simulink model "MCCULLOUGH_Andrew_Proj4_simulink"  (R2018b)
settings: Solver=FixedStepDiscrete  StartTime=0.0  StopTime=0.1  FixedStep=1e-7  RelTol=1e-3
libraries: powerlib x20, simulink x1
settings Model: Creator=Andrew McCullough  LastModifiedBy=Andrew McCullough

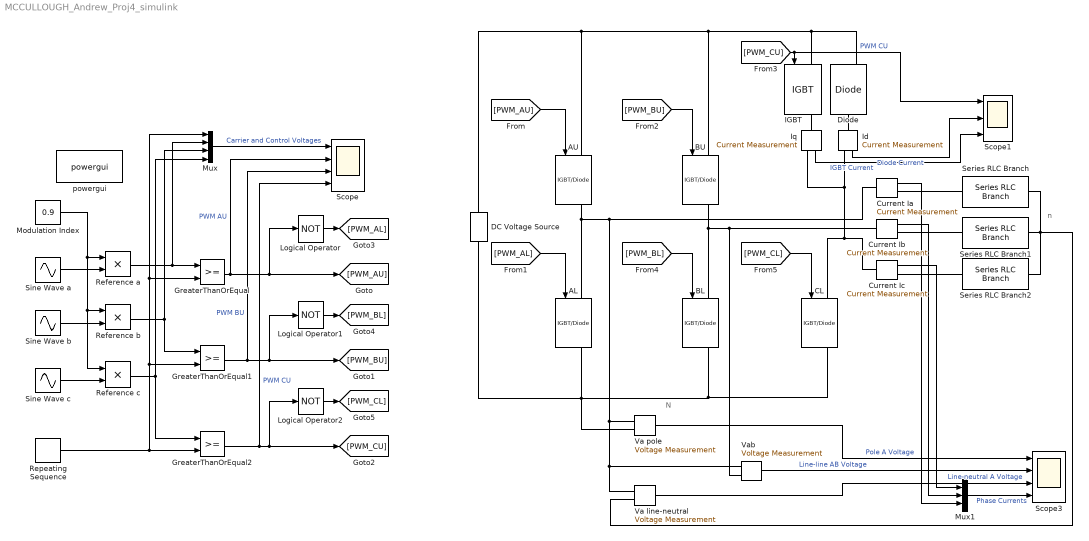
== system MCCULLOUGH_Andrew_Proj4_simulink ==
  note: n
  note: N
  AL : powerlib/Power Electronics/IGBT//Diode  Ron=1e-3  Rs=1e5  Cs=inf  Measurements=on
  AU : powerlib/Power Electronics/IGBT//Diode  Ron=1e-3  Rs=1e5  Cs=inf  Measurements=on
  BL : powerlib/Power Electronics/IGBT//Diode  Ron=1e-3  Rs=1e5  Cs=inf  Measurements=on
  BU : powerlib/Power Electronics/IGBT//Diode  Ron=1e-3  Rs=1e5  Cs=inf  Measurements=on
  CL : powerlib/Power Electronics/IGBT//Diode  Ron=1e-3  Rs=1e5  Cs=inf  Measurements=on
  Current Ia : powerlib/Measurements/Current Measurement  PhasorSimulation=off  OutputType=Complex  PSBequivalent=0
  Current Ib : powerlib/Measurements/Current Measurement  PhasorSimulation=off  OutputType=Complex  PSBequivalent=0
  Current Ic : powerlib/Measurements/Current Measurement  PhasorSimulation=off  OutputType=Complex  PSBequivalent=0
  DC Voltage Source : powerlib/Electrical Sources/DC Voltage Source  Amplitude=400  Measurements=None
  Diode : powerlib/Power Electronics/Diode  Ron=0.001  Lon=0  Vf=0.8  IC=0  UseSnubber=0  Rs=500  Cs=250e-9  Measurements=on
  GreaterThanOrEqual : RelationalOperator  OutDataTypeStr=boolean  RndMeth=Simplest
  GreaterThanOrEqual1 : RelationalOperator  OutDataTypeStr=boolean  RndMeth=Simplest
  GreaterThanOrEqual2 : RelationalOperator  OutDataTypeStr=boolean  RndMeth=Simplest
  IGBT : powerlib/Power Electronics/IGBT  Ron=0.001  Lon=0  Vf=1  Tf=1e-6  Tt=2e-6  IC=0  Rs=1e5  Cs=inf  Measurements=on
  Id : powerlib/Measurements/Current Measurement  PhasorSimulation=off  OutputType=Complex  PSBequivalent=0
  Iq : powerlib/Measurements/Current Measurement  PhasorSimulation=off  OutputType=Complex  PSBequivalent=0
  Logical Operator : Logic  Operator=NOT  AllPortsSameDT=off  OutDataTypeStr=boolean
  Logical Operator1 : Logic  Operator=NOT  AllPortsSameDT=off  OutDataTypeStr=boolean
  Logical Operator2 : Logic  Operator=NOT  AllPortsSameDT=off  OutDataTypeStr=boolean
  Modulation Index : Constant  Value=0.9
  Mux : Mux
  Mux1 : Mux  Inputs=3
  Reference a : Product
  Reference b : Product
  Reference c : Product
  Repeating Sequence : simulink/Sources/Repeating Sequence  rep_seq_t=[0 ((1/2)*(1/15000)) (1/15000)]  rep_seq_y=[-1 1 -1]
  Scope : Scope  NumInputPorts=4
  Scope1 : Scope  NumInputPorts=3
  Scope3 : Scope  NumInputPorts=4
  Series RLC Branch : powerlib/Elements/Series RLC Branch  LConnTagsString=__new0  RConnTagsString=__new0  BranchType=RL  Resistance=.3  Inductance=0.2e-3  SetiL0=off  InitialCurrent=0  Capacitance=0  Setx0=off  InitialVoltage=0  Measurements=None
  Series RLC Branch1 : powerlib/Elements/Series RLC Branch  LConnTagsString=__new0  RConnTagsString=__new0  BranchType=RL  Resistance=.3  Inductance=0.2e-3  SetiL0=off  InitialCurrent=0  Capacitance=0  Setx0=off  InitialVoltage=0  Measurements=None
  Series RLC Branch2 : powerlib/Elements/Series RLC Branch  LConnTagsString=__new0  RConnTagsString=__new0  BranchType=RL  Resistance=.3  Inductance=0.2e-3  SetiL0=off  InitialCurrent=0  Capacitance=0  Setx0=off  InitialVoltage=0  Measurements=None
  Sine Wave a : Sin  Frequency=2*100*pi  SampleTime=0
  Sine Wave b : Sin  Frequency=2*100*pi  Phase=120*(pi/180)  SampleTime=0
  Sine Wave c : Sin  Frequency=2*100*pi  Phase=-120*(pi/180)  SampleTime=0
  Va line-neutral : powerlib/Measurements/Voltage Measurement  PhasorSimulation=off  OutputType=Complex  PSBequivalent=0
  Va pole : powerlib/Measurements/Voltage Measurement  PhasorSimulation=off  OutputType=Complex  PSBequivalent=0
  Vab : powerlib/Measurements/Voltage Measurement  PhasorSimulation=off  OutputType=Complex  PSBequivalent=0
  powergui : powerlib/powergui  Priority=1  SimulationMode=Discrete  SampleTime=1e-7  frequency=60  Iterations=50  frequencyindice=0  Pbase=100e6  ErrMax=1e-4  UnitsV=kV  UnitsW=MW  buscounter=0  FunctionMessages=off  echomessages=off  EnableUseOfTLC=off  CurrentSourceSwitches=off  DisableSnubberDevices=off  DisableRonSwitches=off  DisableVfSwitches=off  DisplayEquations=off  SolverType=Tustin/Backward Euler (TBE)  Interpol=off  ExternalGateDelay=off  methode=off  Ts=100  x0status=blocks  SPID=off  SwTol=0  HookPort=off  RestoreLinks=warning  ResistiveCurrentMeasurement=off  Frange=[0:2:500]  Ylog=off  Xlog=on  ShowGrid=off  save=off  variable=ZData  structure=0  ZoomFFT=off  StartTime=0.0  cycles=1  DisplayStyle=1  fundamental=60  FreqAxis=off  MaxFrequency=1000  frequencyindicesteady=1  RmsSteady=1  display=off
  wires:
  Sine Wave a/1 -> Reference a/2
  Sine Wave b/1 -> Reference b/2
  Sine Wave c/1 -> Reference c/2
  Modulation Index/1 -> Reference a/1, Reference b/1, Reference c/1
  Reference a/1 -> GreaterThanOrEqual/1, Mux/2
  Reference b/1 -> GreaterThanOrEqual1/1, Mux/3
  Reference c/1 -> GreaterThanOrEqual2/1, Mux/4
  Repeating Sequence/1 -> Mux/1, GreaterThanOrEqual/2, GreaterThanOrEqual1/2, GreaterThanOrEqual2/2
  GreaterThanOrEqual2/1 -> Logical Operator2/1, [PWM_CU], Scope/4  "PWM CU"
  GreaterThanOrEqual1/1 -> Logical Operator1/1, [PWM_BU], Scope/3  "PWM BU"
  GreaterThanOrEqual/1 -> [PWM_AU], Logical Operator/1, Scope/2  "PWM AU"
  Logical Operator/1 -> [PWM_AL]
  Logical Operator1/1 -> [PWM_BL]
  Logical Operator2/1 -> [PWM_CL]
  Mux/1 -> Scope/1  "Carrier and Control Voltages"
  [PWM_AU] -> AU/1
  [PWM_BU] -> BU/1
  [PWM_AL] -> AL/1
  [PWM_BL] -> BL/1
  [PWM_CL] -> CL/1
  Va pole/1 -> Scope3/1  "Pole A Voltage"
  Current Ia/1 -> Mux1/3
  Current Ib/1 -> Mux1/2
  Current Ic/1 -> Mux1/1
  Mux1/1 -> Scope3/4  "Phase Currents"
  Vab/1 -> Scope3/2  "Line-line AB Voltage"
  Va line-neutral/1 -> Scope3/3  "Line-neutral A Voltage"
  [PWM_CU] -> Scope1/1, IGBT/1  "PWM CU"
  Id/1 -> Scope1/2  "Diode Current"
  Iq/1 -> Scope1/3  "IGBT Current"
  connections:
  Vab/LConn2 -- Current Ib/LConn1 -- BL/LConn1 -- BU/RConn1
  Current Ia/RConn1 -- Series RLC Branch/LConn1
  Series RLC Branch1/LConn1 -- Current Ib/RConn1
  Series RLC Branch2/LConn1 -- Current Ic/RConn1
  CL/RConn1 -- BL/RConn1 -- AL/RConn1 -- DC Voltage Source/LConn1 -- Va pole/LConn2
  Va pole/LConn1 -- AL/LConn1 -- AU/RConn1 -- Current Ia/LConn1 -- Va line-neutral/LConn1 -- Vab/LConn1
  Series RLC Branch/RConn1 -- Series RLC Branch2/RConn1 -- Series RLC Branch1/RConn1 -- Va line-neutral/LConn2
  DC Voltage Source/RConn1 -- AU/LConn1 -- BU/LConn1 -- Diode/RConn1 -- IGBT/LConn1
  Current Ic/LConn1 -- Iq/RConn1 -- Id/RConn1 -- CL/LConn1
  Iq/LConn1 -- IGBT/RConn1
  Id/LConn1 -- Diode/LConn1
